simulink model "combined_electrolyzer"  (R2023a)
settings: Solver=FixedStepAuto  StartTime=0.0  StopTime=3600  FixedStep=1  RelTol=1e-3
settings Model: Creator=Anupp  LastModifiedBy=Anupp
settings ModelReferenceCC: EnableRefExpFcnMdlSchedulingChecks=on

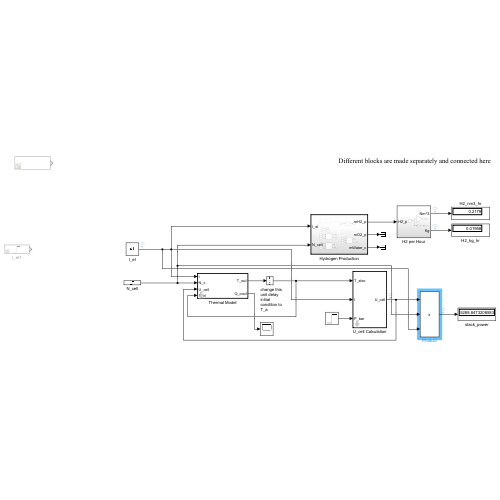
[thumbnail: Simulink's stored preview of the top-level diagram]
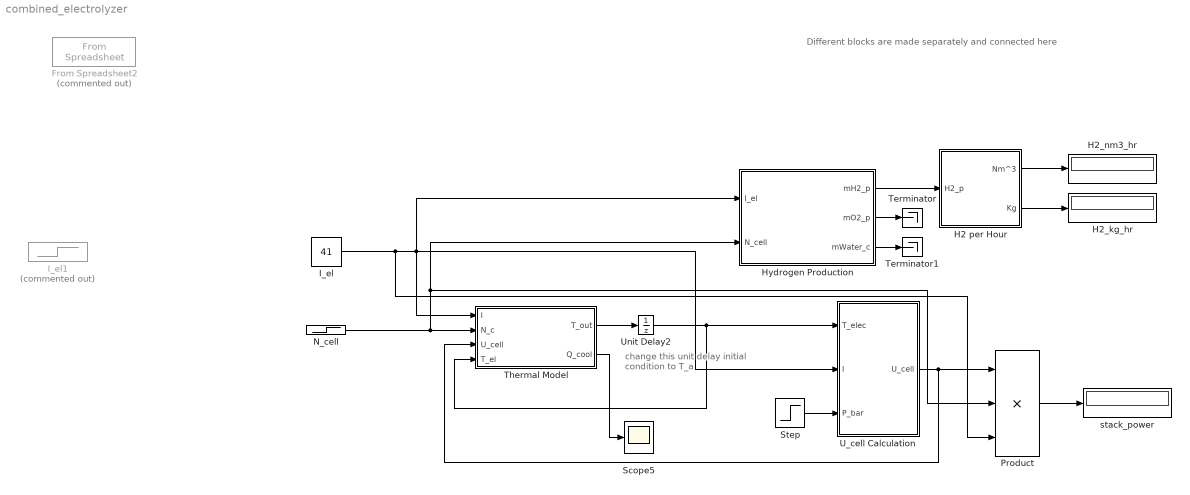
== system combined_electrolyzer ==
  note: Different blocks are made separately and connected here
  note: change this unit delay initial condition to T_a
  From Spreadsheet2 : FromSpreadsheet  Commented=on  FileName=E:\tintan\Matlab alakaline electrolysis new\data test\down_dynamic_halved.csv  SheetName=down_dynamic_halved
  H2 per Hour : Subsystem
  H2_kg_hr : Display
  H2_nm3_hr : Display
  Hydrogen Production : Subsystem  TreatAsAtomicUnit=on
  I_el : Constant  Value=41
  I_el1 : Step  Commented=on  Time=0  After=125  SampleTime=0
  N_cell : Step  Time=0  After=75  SampleTime=0
  Product : Product  Inputs=3
  Scope5 : Scope
  Step : Step  Time=0  After=9.44  SampleTime=0
  Terminator : Terminator
  Terminator1 : Terminator
  Thermal Model : Subsystem  TreatAsAtomicUnit=on  mask{E_tn=1.476, T_a=298, R_t=0.167, C_t=11, T_nominal=345}
      mask prompts: E_tn "Thermo-neutral voltage (E_tn)"; T_a "Ambient Temperature (kelvin)"; R_t "Thermal Resistance"; C_t "Thermal Capacitance"; T_nominal "Nominal Temperature (kelvin)"
  U_cell Calculation : Subsystem  TreatAsAtomicUnit=on  mask{A=2082, r1=5.463162, r2=-0.044073, t1=1197.525356, t2=-38432.6689, t3=1322570.138, s=0.161, C=0.25}
      mask prompts: A "Area"; r1 "r1 for U_ohm"; r2 "r2 for U_ohm"; t1 "t1 for U_act"; t2 "t2 for U_act"; t3 "t3 for U_act"; s "s for U_act"; C "Concentration by weight (decimal)"
      mask DialogControl DescTextVar Prompt: Put all values in terms in Metres only or Cm only. Also check if U_act variables is for Log or Ln (change accordingly inside the mask). Also, use concentration value as decimal (for eg. use 0.25, don't use 25 percent).
  Unit Delay2 : UnitDelay  InitialCondition=298  SampleTime=-1  HasFrameUpgradeWarning=on
  stack_power : Display
  wires:
  Thermal Model/1(T_out) -> Unit Delay2/1
  U_cell Calculation/1(U_cell) -> Thermal Model/3(U_cell), Product/1
  Unit Delay2/1 -> Thermal Model/4(T_el), U_cell Calculation/1(T_elec)
  I_el/1 -> Product/3, U_cell Calculation/2(I), Thermal Model/1(I), Hydrogen Production/1(I_el)
  N_cell/1 -> Hydrogen Production/2(N_cell), Product/2, Thermal Model/2(N_c)
  Thermal Model/2(Q_cool) -> Scope5/1
  Step/1 -> U_cell Calculation/3(P_bar)
  Hydrogen Production/2(mO2_p) -> Terminator/1
  Hydrogen Production/3(mWater_c) -> Terminator1/1
  Hydrogen Production/1(mH2_p) -> H2 per Hour/1(H2_p)
  H2 per Hour/1(Nm^3) -> H2_nm3_hr/1
  H2 per Hour/2(Kg) -> H2_kg_hr/1
  Product/1 -> stack_power/1

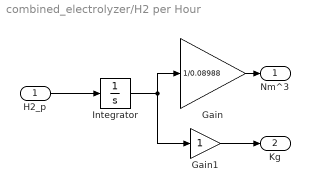
== system combined_electrolyzer/H2 per Hour ==
  H2_p : Inport
  Gain : Gain  Gain=1/0.08988
  Gain1 : Gain
  Integrator : Integrator
  Nm^3 : Outport
  Kg : Outport  Port=2
  wires:
  Integrator/1 -> Gain1/1, Gain/1
  H2_p/1 -> Integrator/1
  Gain/1 -> Nm^3/1
  Gain1/1 -> Kg/1

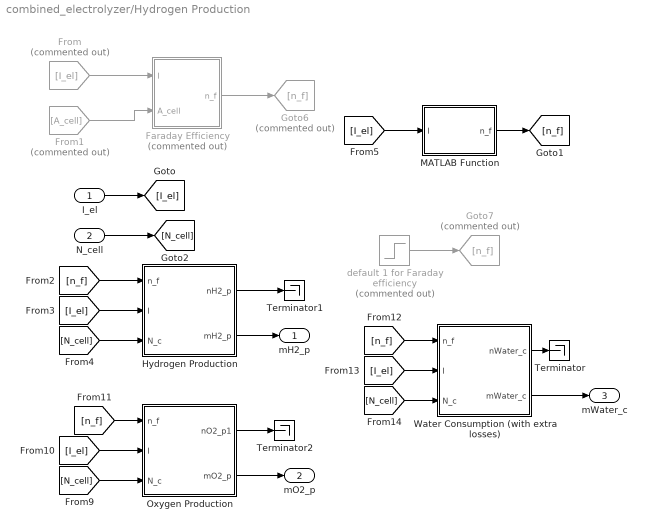
== system combined_electrolyzer/Hydrogen Production ==
  I_el : Inport
  N_cell : Inport  Port=2
  Faraday Efficiency : Subsystem  Commented=on  mask{a1=0, a2=0, a3=0}
      mask DialogControl DescTextVar Prompt: Define Faraday's efficiency parameters for alkaline electrolyser
  From : From  Commented=on  GotoTag=I_el
  From1 : From  Commented=on  GotoTag=A_cell
  Goto6 : Goto  Commented=on  GotoTag=n_f
  Goto7 : Goto  Commented=on  GotoTag=n_f
  Hydrogen Production : Subsystem
  MATLAB Function : MATLAB Function  TreatAsAtomicUnit=on
  Oxygen Production : Subsystem
  Terminator : Terminator
  Terminator1 : Terminator
  Terminator2 : Terminator
  Water Consumption (with extra losses) : Subsystem
  default 1 for Faraday efficiency : Step  Commented=on  Time=0  After=0.86  SampleTime=0
  mH2_p : Outport
  mO2_p : Outport  Port=2
  mWater_c : Outport  Port=3
  wires:
  From1/1 -> Faraday Efficiency/2(A_cell)
  From/1 -> Faraday Efficiency/1(I)
  [n_f] -> Hydrogen Production/1(n_f)
  [I_el] -> Water Consumption (with extra losses)/2(I)
  Hydrogen Production/2(mH2_p) -> mH2_p/1
  I_el/1 -> [I_el]
  [n_f] -> Oxygen Production/1(n_f)
  Water Consumption (with extra losses)/2(mWater_c) -> mWater_c/1
  [I_el] -> Oxygen Production/2(I)
  [N_cell] -> Oxygen Production/3(N_c)
  [N_cell] -> Hydrogen Production/3(N_c)
  Oxygen Production/2(mO2_p) -> mO2_p/1
  [I_el] -> Hydrogen Production/2(I)
  Faraday Efficiency/1(n_f) -> Goto6/1
  [N_cell] -> Water Consumption (with extra losses)/3(N_c)
  [n_f] -> Water Consumption (with extra losses)/1(n_f)
  Water Consumption (with extra losses)/1(nWater_c) -> Terminator/1
  Hydrogen Production/1(nH2_p) -> Terminator1/1
  Oxygen Production/1(nO2_p1) -> Terminator2/1
  default 1 for Faraday efficiency/1 -> Goto7/1
  [I_el] -> MATLAB Function/1(I)
  MATLAB Function/1(n_f) -> [n_f]
  N_cell/1 -> [N_cell]

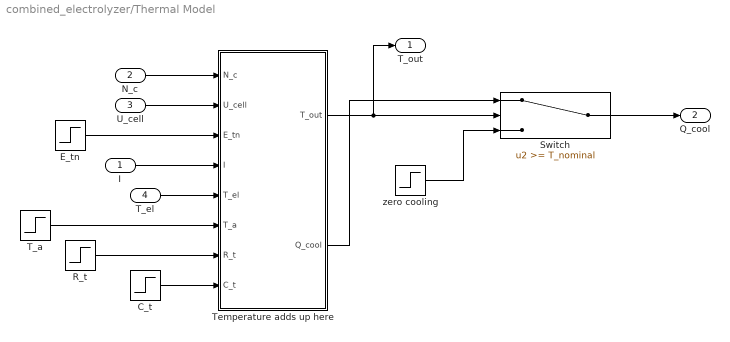
== system combined_electrolyzer/Thermal Model ==
  I : Inport
  N_c : Inport  Port=2
  U_cell : Inport  Port=3
  T_el : Inport  Port=4
  C_t : Step  Time=0  After=C_t  SampleTime=0
  E_tn : Step  Time=0  After=E_tn  SampleTime=0
  R_t : Step  Time=0  After=R_t  SampleTime=0
  Switch : Switch  Threshold=T_nominal  SaturateOnIntegerOverflow=off  InputSameDT=off
  T_a : Step  Time=0  After=T_a  SampleTime=0
  Temperature adds up here : Subsystem
  zero cooling : Step  Time=0  After=0  SampleTime=0
  T_out : Outport
  Q_cool : Outport  Port=2
  wires:
  C_t/1 -> Temperature adds up here/8(C_t)
  I/1 -> Temperature adds up here/4(I)
  E_tn/1 -> Temperature adds up here/3(E_tn)
  U_cell/1 -> Temperature adds up here/2(U_cell)
  N_c/1 -> Temperature adds up here/1(N_c)
  T_a/1 -> Temperature adds up here/6(T_a)
  R_t/1 -> Temperature adds up here/7(R_t)
  T_el/1 -> Temperature adds up here/5(T_el)
  Temperature adds up here/1(T_out) -> T_out/1, Switch/2
  zero cooling/1 -> Switch/3
  Switch/1 -> Q_cool/1
  Temperature adds up here/2(Q_cool) -> Switch/1

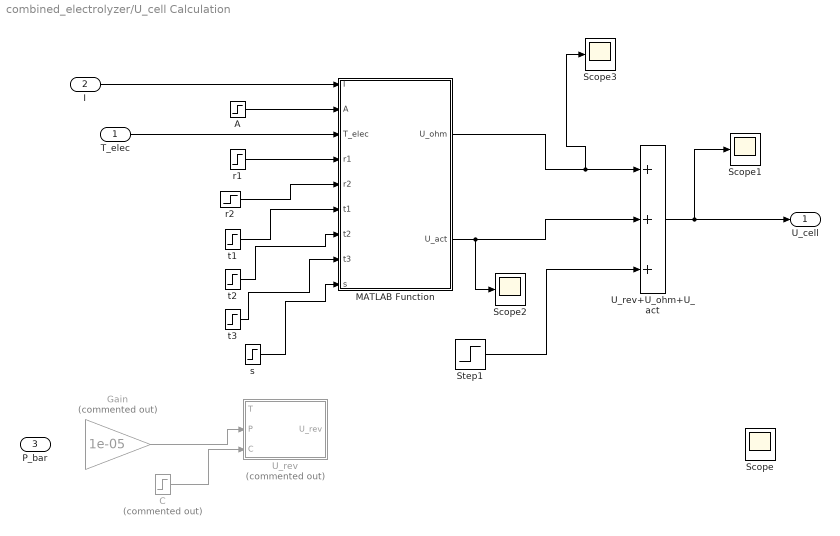
== system combined_electrolyzer/U_cell Calculation ==
  T_elec : Inport
  I : Inport  Port=2
  P_bar : Inport  Port=3
  A : Step  Time=0  After=A  SampleTime=0
  C : Step  Commented=on  Time=0  After=C  SampleTime=0
  Gain : Gain  Commented=on  Gain=1e-05
  MATLAB Function : MATLAB Function  TreatAsAtomicUnit=on
  Scope{,1..3} (4 alike) : Scope
  Step1 : Step  Time=0  After=1.2  SampleTime=0
  U_rev : MATLAB Function  Commented=on  TreatAsAtomicUnit=on
  U_rev+U_ohm+U_act : Sum  Inputs=+++
  r1 : Step  Time=0  After=r1  SampleTime=0
  r2 : Step  Time=0  After=r2  SampleTime=0
  s : Step  Time=0  After=s  SampleTime=0
  t1 : Step  Time=0  After=t1  SampleTime=0
  t2 : Step  Time=0  After=t2  SampleTime=0
  t3 : Step  Time=0  After=t3  SampleTime=0
  U_cell : Outport
  wires:
  T_elec/1 -> MATLAB Function/3(T_elec)
  U_rev+U_ohm+U_act/1 -> U_cell/1, Scope1/1
  C/1 -> U_rev/3(C)
  r1/1 -> MATLAB Function/4(r1)
  r2/1 -> MATLAB Function/5(r2)
  t1/1 -> MATLAB Function/6(t1)
  t2/1 -> MATLAB Function/7(t2)
  t3/1 -> MATLAB Function/8(t3)
  s/1 -> MATLAB Function/9(s)
  I/1 -> MATLAB Function/1(I)
  A/1 -> MATLAB Function/2(A)
  MATLAB Function/2(U_act) -> Scope2/1, U_rev+U_ohm+U_act/2
  MATLAB Function/1(U_ohm) -> Scope3/1, U_rev+U_ohm+U_act/1
  Gain/1 -> U_rev/2(P)
  Step1/1 -> U_rev+U_ohm+U_act/3

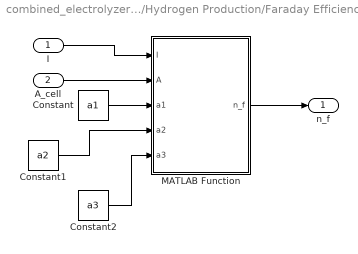
== system combined_electrolyzer/Hydrogen Production/Faraday Efficiency ==
  I : Inport
  A_cell : Inport  Port=2
  Constant : Constant  Value=a1
  Constant1 : Constant  Value=a2
  Constant2 : Constant  Value=a3
  MATLAB Function : MATLAB Function  TreatAsAtomicUnit=on
  n_f : Outport
  wires:
  MATLAB Function/1(n_f) -> n_f/1
  Constant2/1 -> MATLAB Function/5(a3)
  Constant1/1 -> MATLAB Function/4(a2)
  A_cell/1 -> MATLAB Function/2(A)
  I/1 -> MATLAB Function/1(I)
  Constant/1 -> MATLAB Function/3(a1)

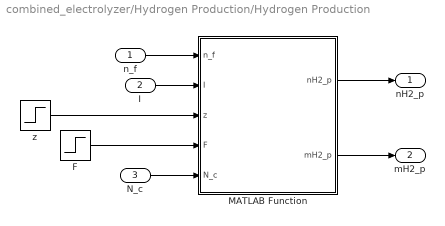
== system combined_electrolyzer/Hydrogen Production/Hydrogen Production ==
  n_f : Inport
  I : Inport  Port=2
  N_c : Inport  Port=3
  F : Step  Time=0  After=96485  SampleTime=0
  MATLAB Function : MATLAB Function  TreatAsAtomicUnit=on
  z : Step  Time=0  After=2  SampleTime=0
  nH2_p : Outport
  mH2_p : Outport  Port=2
  wires:
  n_f/1 -> MATLAB Function/1(n_f)
  I/1 -> MATLAB Function/2(I)
  MATLAB Function/2(mH2_p) -> mH2_p/1
  N_c/1 -> MATLAB Function/5(N_c)
  F/1 -> MATLAB Function/4(F)
  z/1 -> MATLAB Function/3(z)
  MATLAB Function/1(nH2_p) -> nH2_p/1

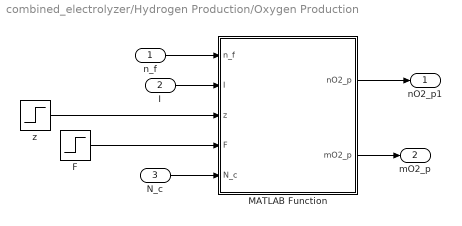
== system combined_electrolyzer/Hydrogen Production/Oxygen Production ==
  n_f : Inport
  I : Inport  Port=2
  N_c : Inport  Port=3
  F : Step  Time=0  After=96485  SampleTime=0
  MATLAB Function : MATLAB Function  TreatAsAtomicUnit=on
  z : Step  Time=0  After=2  SampleTime=0
  nO2_p1 : Outport
  mO2_p : Outport  Port=2
  wires:
  n_f/1 -> MATLAB Function/1(n_f)
  I/1 -> MATLAB Function/2(I)
  MATLAB Function/2(mO2_p) -> mO2_p/1
  N_c/1 -> MATLAB Function/5(N_c)
  MATLAB Function/1(nO2_p) -> nO2_p1/1
  F/1 -> MATLAB Function/4(F)
  z/1 -> MATLAB Function/3(z)

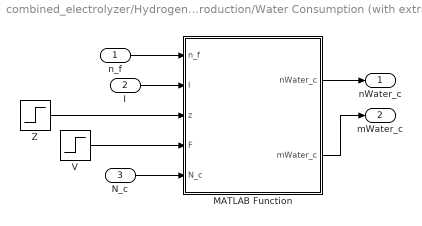
== system combined_electrolyzer/Hydrogen Production/Water Consumption (with extra losses) ==
  n_f : Inport
  I : Inport  Port=2
  N_c : Inport  Port=3
  MATLAB Function : MATLAB Function  TreatAsAtomicUnit=on
  V : Step  Time=0  After=96485  SampleTime=0
  Z : Step  Time=0  After=2  SampleTime=0
  nWater_c : Outport
  mWater_c : Outport  Port=2
  wires:
  n_f/1 -> MATLAB Function/1(n_f)
  I/1 -> MATLAB Function/2(I)
  MATLAB Function/2(mWater_c) -> mWater_c/1
  N_c/1 -> MATLAB Function/5(N_c)
  MATLAB Function/1(nWater_c) -> nWater_c/1
  Z/1 -> MATLAB Function/3(z)
  V/1 -> MATLAB Function/4(F)

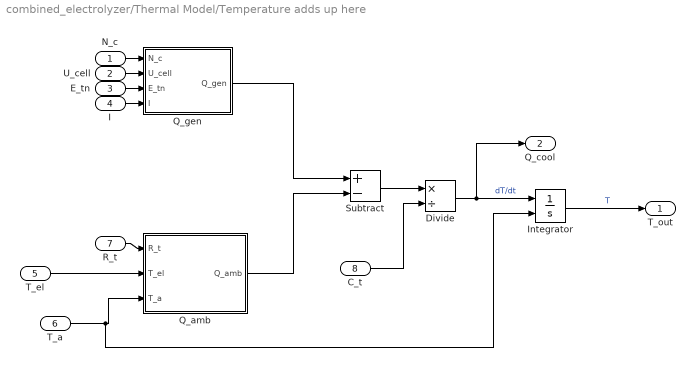
== system combined_electrolyzer/Thermal Model/Temperature adds up here ==
  N_c : Inport
  U_cell : Inport  Port=2
  E_tn : Inport  Port=3
  I : Inport  Port=4
  T_el : Inport  Port=5
  T_a : Inport  Port=6
  R_t : Inport  Port=7
  C_t : Inport  Port=8
  Divide : Product  Inputs=*/
  Integrator : Integrator  InitialConditionSource=external  LimitOutput=on  UpperSaturationLimit=T_nominal
  Q_amb : MATLAB Function  TreatAsAtomicUnit=on
  Q_gen : MATLAB Function  TreatAsAtomicUnit=on
  Subtract : Sum  Inputs=+-
  T_out : Outport
  Q_cool : Outport  Port=2
  wires:
  Q_gen/1(Q_gen) -> Subtract/1
  Q_amb/1(Q_amb) -> Subtract/2
  Integrator/1 -> T_out/1  "T"
  Divide/1 -> Q_cool/1, Integrator/1  "dT/dt"
  C_t/1 -> Divide/2
  R_t/1 -> Q_amb/1(R_t)
  Subtract/1 -> Divide/1
  N_c/1 -> Q_gen/1(N_c)
  E_tn/1 -> Q_gen/3(E_tn)
  I/1 -> Q_gen/4(I)
  U_cell/1 -> Q_gen/2(U_cell)
  T_a/1 -> Integrator/2, Q_amb/3(T_a)
  T_el/1 -> Q_amb/2(T_el)

== matlab function combined_electrolyzer/Hydrogen Production/Water Consumption (with extra losses)/MATLAB Function ==
  data: nWater_c output; n_f input; mWater_c output; I input; z input; F input; N_c input
function [nWater_c,mWater_c] = fcn(n_f,I,z,F,N_c)

nWater_c = 1.25 * n_f * I * N_c / (z * F);

mWater_c = 18.015 * 1e-3 * nWater_c;

end

== matlab function combined_electrolyzer/Thermal Model/Temperature adds up here/Q_gen ==
  data: N_c input; Q_gen output; U_cell input; E_tn input; I input
function Q_gen = fcn(N_c,U_cell,E_tn,I)

Q_gen = N_c * (U_cell - E_tn) * I;

end

== matlab function combined_electrolyzer/U_cell Calculation/MATLAB Function ==
  data: I input; U_ohm output; A input; T_elec input; r1 input; r2 input; t1 input; t2 input; t3 input; s input; U_act output
function [U_ohm, U_act] = fcn(I,A,T_elec,r1,r2,t1,t2,t3,s)

T = T_elec-273;

i = I/A;

U_ohm = (r1 + r2*T)*i;

U_act = s*log((t1 + t2/T + t3/(T^2))*i + 1);

end

== matlab function combined_electrolyzer/Thermal Model/Temperature adds up here/Q_amb ==
  data: R_t input; Q_amb output; T_el input; T_a input
function Q_amb = fcn(R_t,T_el,T_a)

Q_amb = (T_el - T_a)/R_t;

end

== matlab function combined_electrolyzer/U_cell Calculation/U_rev ==
  data: T input; U_rev output; P input; C input
function U_rev = fcn(T,P,C)
% T = 398;
% P = 9.44;
% C = 0.25;
R = 8.3144598; %J. mol-1
z = 2; %of hydrogen is used, don't know why oxygen is not used
F = 96485; %Faradays constant C/mol
M = ((312500/17533)*C)/(1-C); %molality

U_0rev = 1.5184-1.5421*10^(-3)*T+9.526*10^(-5)*T*log(T)+9.84*10^(-8)*(T)^2;

a = -0.0151*M - 1.6788*10^(-3)*(M^2)+2.2588*10^(-5)*(M^3);
b = 1-1.2062*10^(-3)*M+5.6024*10^(-4)*(M^2)-7.8228*10^(-6)*(M^3);
P_vH2O = 10^(5.1962-(1730.63/(233.426+T-273)));
%P_vH2O = exp(81.6179 - 7699.68/T - 10.9*log(T) + 9.5891 * 10^(-3) * T);

P_vKOH = exp(2.302*a+b*log(P_vH2O));

a_H2O_KOH = exp(-0.05192*M+0.003302*(M^2)+((3.177*M-2.131*(M^2))/T));

U_rev = U_0rev + ((R*T)/(z*F))*log10(((P-P_vKOH)*((P-P_vKOH)^0.5))/(a_H2O_KOH));

end

== matlab function combined_electrolyzer/Hydrogen Production/MATLAB Function ==
  data: I input; n_f output
function n_f = fcn(I)

n_f = -2.4415e-09.*I.^4 + 1.5597e-06.*I.^3 - 3.6911e-04.*I.^2 + 0.03889.*I - 0.90529;

end

== matlab function combined_electrolyzer/Hydrogen Production/Faraday Efficiency/MATLAB Function ==
  data: I input; n_f output; A input; a1 input; a2 input; a3 input
function n_f = fcn(I,A,a1,a2,a3)

n_f = a1 .* exp(a2/(I/A) + a3/(I/A)^2);

end

== matlab function combined_electrolyzer/Hydrogen Production/Hydrogen Production/MATLAB Function ==
  data: nH2_p output; n_f input; mH2_p output; I input; z input; F input; N_c input
function [nH2_p,mH2_p] = fcn(n_f,I,z,F,N_c)

nH2_p = n_f * I * N_c / (z * F);
mH2_p = 2.016 * 1e-3 * nH2_p; 

end

== matlab function combined_electrolyzer/Hydrogen Production/Oxygen Production/MATLAB Function ==
  data: nO2_p output; n_f input; mO2_p output; I input; z input; F input; N_c input
function [nO2_p,mO2_p] = fcn(n_f,I,z,F,N_c)

nO2_p = 0.5 * n_f * I * N_c / (z * F);

mO2_p = 32 * 1e-3 * nO2_p;

end
